simulink model "vidcap_webcam"  (R2018a)
settings: Solver=FixedStepAuto  StartTime=0.0  StopTime=inf  RelTol=1e-3  EnableMultiTasking=on
undefined symbols (not defined in the file): Rec, SDTV, videoinput
libraries: embdlinuxlib x3, simulink x3, visiontextngfix x2, visionstatistics x1, visionconversions x1, imaqlib x1, visionanalysis x1
settings Model: Creator=migue  LastModifiedBy=migue
settings SolverCC: PositivePriorityOrder=on
settings OptimizationCC: EnhancedBackFolding=on  PassReuseOutputArgsAs=Individual arguments  MaxStackSize=64  OptimizeBlockOrder=speed  DifferentSizesBufferReuse=on  OptimizationCustomize=off
settings DebuggingCC: ParameterTunabilityLossMsg=error
settings HardwareCC: ProdBitPerPointer=32  ProdBitPerSizeT=32  ProdBitPerPtrDiffT=32  ProdLargestAtomicInteger=Long  ProdLargestAtomicFloat=Double  ProdWordSize=32  ProdHWDeviceType=ARM Compatible->ARM Cortex
settings SFSimCC: MATLABDynamicMemAlloc=off
settings RTWCC: SystemTargetFile=ert.tlc  HardwareBoard=Raspberry Pi  TLCOptions="-aInlineSetEventsForThisBaseRateFcn=TLC_FALSE -aSuppressMultiTaskScheduler=TLC_FALSE  -aRateBasedStepFcn=0"  TemplateMakefile=ert_default_tmf  GenerateReport=on  Toolchain=GNU GCC Raspberry Pi  BuildConfiguration=Faster Runs  IncludeHyperlinkInReport=on  LaunchReport=on  GenerateTraceInfo=on  GenerateTraceReport=on  GenerateTraceReportSl=on  GenerateTraceReportSf=on  GenerateTraceReportEml=on
settings CodeAppCC: ForceParamTrailComments=on  IgnoreCustomStorageClasses=off  OperatorAnnotations=on  SimulinkDataObjDesc=on  SFDataObjDesc=on  InsertBlockDesc=on
settings ERTTargetCC: SupportVariableSizeSignals=on

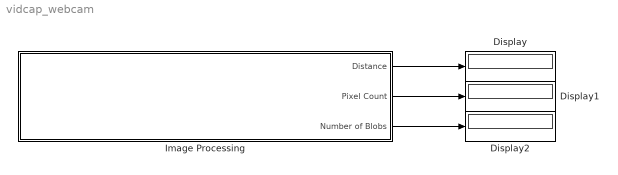
== system vidcap_webcam ==
  Display : Display
  Display1 : Display
  Display2 : Display
  "Image Processing " : Subsystem
  wires:
  "Image Processing "/1(Distance) -> Display/1
  "Image Processing "/2(Pixel Count) -> Display1/1
  "Image Processing "/3(Number of Blobs) -> Display2/1

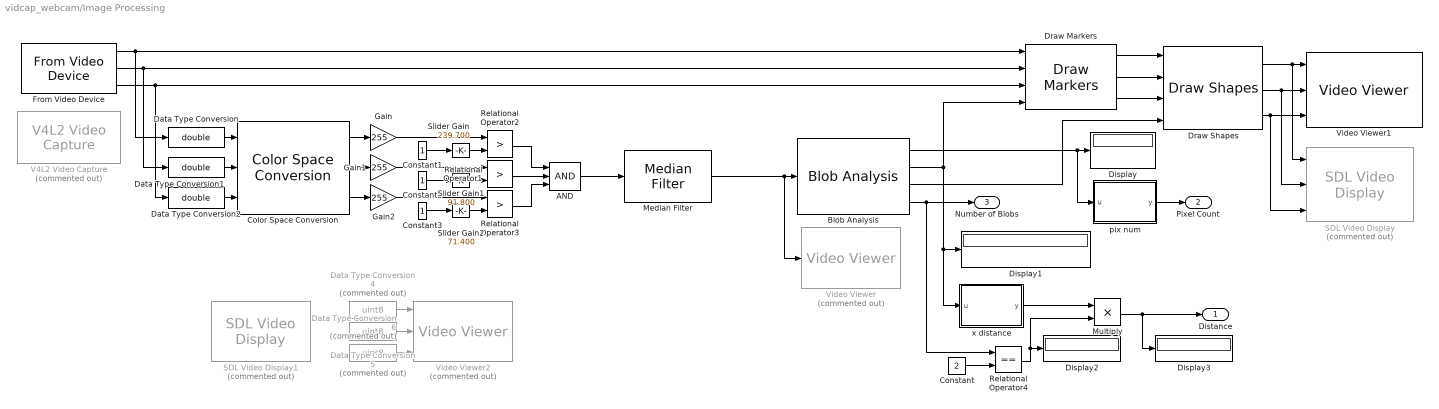
== system vidcap_webcam/Image Processing  ==
  AND : Logic  Inputs=3  IconShape=distinctive  AllPortsSameDT=off  OutDataTypeStr=boolean
  Blob Analysis : visionstatistics/Blob Analysis  Tag=vipblks_row_conv  area=on  centroid=on  bBox=on  majorAxis=off  minorAxis=off  angle=off  eccentricity=off  equivDiameterSq=off  extent=off  perimeter=off  maxBlobs=2  warnIfNumBlobsExceeded=on  isCount=on  useMinArea=on  minArea=2500  useMaxArea=off  maxArea=intmax('uint32')  excludeBorderBlob=off  outDT=double  isOutVarDim=off  isFill=on  fillValues=-1  conn=8  isLabel=off  outputMode=Binary point scaling  outputWordLength=32  outputFracLength=16  firstCoeffMode=Binary point scaling  firstCoeffWordLength=16  firstCoeffFracLength=14  secondCoeffMode=Binary point scaling  secondCoeffWordLength=32  secondCoeffFracLength=16  accumMode=Binary point scaling  accumWordLength=32  accumFracLength=0  prodOutputMode=Binary point scaling  prodOutputWordLength=32  prodOutputFracLength=16  roundingMode=Floor  overflowMode=off
      settings: SourceProductName=Computer Vision System Toolbox
  Color Space Conversion : visionconversions/Color Space  Conversion  conversion=Obsolete  conversionActive=R'G'B' to HSV  wp_str=D65  rec=Rec. 601 (SDTV)  sys=1125/60/2:1  imagePorts=Separate color signals
      settings: SourceProductName=Computer Vision System Toolbox
  Constant : Constant  Value=2
  Constant1 : Constant  OutDataTypeStr=uint8
  Constant2 : Constant  OutDataTypeStr=uint8
  Constant3 : Constant  OutDataTypeStr=uint8
  Data Type Conversion : DataTypeConversion  OutDataTypeStr=double  RndMeth=Simplest  LockScale=on
  Data Type Conversion1 : DataTypeConversion  OutDataTypeStr=double  RndMeth=Simplest  LockScale=on
  Data Type Conversion2 : DataTypeConversion  OutDataTypeStr=double  RndMeth=Simplest  LockScale=on
  Data Type Conversion4 : DataTypeConversion  Commented=on  OutDataTypeStr=uint8
  Data Type Conversion5 : DataTypeConversion  Commented=on  OutDataTypeStr=uint8
  Data Type Conversion6 : DataTypeConversion  Commented=on  OutDataTypeStr=uint8
  Display{,1..3} (4 alike) : Display
  Draw Markers : visiontextngfix/Draw Markers  shape=X-mark  size=5  fill=off  fillClrSource=Specify via dialog  display=White  intensity=200  color=[200 255 100]  opacity=0.6  viewport=Entire image  antialiasing=off  inType=Obsolete  imagePorts=Separate color signals  prodOutputMode=Binary point scaling  prodOutputWordLength=32  prodOutputFracLength=14  memoryMode=Specify word length  memoryWordLength=16  memoryFracLength=15  roundingMode=Floor  overflowMode=off
      settings: SourceProductName=Computer Vision System Toolbox  SourceProductBaseCode=VP
  Draw Shapes : visiontextngfix/Draw Shapes  shape=Rectangles  fill=off  lineWidth=3  fillClrSource=Specify via dialog  display=White  intensity=200  color=[200 255 100]  opacity=0.6  viewport=Entire image  antialiasing=off  inType=Obsolete  imagePorts=Separate color signals  prodOutputMode=Binary point scaling  prodOutputWordLength=32  prodOutputFracLength=14  memoryMode=Specify word length  memoryWordLength=16  memoryFracLength=15  roundingMode=Floor  overflowMode=off
      settings: SourceProductName=Computer Vision System Toolbox
  From Video Device : imaqlib/From Video Device  DeviceMenu=winvideo 1 (HD WebCam)  Device=winvideo 1 (HD WebCam)  ObjConstructor=videoinput('winvideo', 1)  VideoFormatMenu=MJPG_1280x720  VideoFormat=MJPG_1280x720  VideoSource=input1  ROIPosition=[0 0 480 640]  EnableHWTrigger=off  TriggerConfiguration=winvideo 1 (HD WebCam)  SampleTime=1/30  OutputPortsMode=Separate color signals  DataType=single  CanDoHWTrigger=no  ReturnedColorSpace=rgb  BlockHandle=250.0001  ROIWidth=640  ROIHeight=480  ROIColumn=0  ROIRow=0  EngXMLPath=C:\Program Files\MATLAB\R2018a\toolbox\imaq\imaq\private  DevXMLPath=C:\ProgramData\MATLAB\SupportPackages\R2018a\toolbox\imaq\supportpackages\genericvideo\adaptor\win64  EngLibPath=C:\Program Files\MATLAB\R2018a\toolbox\imaq\imaqblks\imaqmex\win64  ColorSpace=rgb  BayerSensorAlignment=grbg
      settings: SourceProductName=Image Acquisition Toolbox
  Gain : Gain  Gain=255
  Gain1 : Gain  Gain=255
  Gain2 : Gain  Gain=255
  Median Filter : visionanalysis/Median Filter  nghbood=[5 5]  outSize=Same as input port I  padType=Constant  padSrc=Specify via dialog  padVal=0  roundingMode=Floor  overflowMode=off
      settings: SourceProductName=Computer Vision System Toolbox  SourceProductBaseCode=VP
  Multiply : Product  OutDataTypeStr=double  LockScale=on
  Relational Operator1 : RelationalOperator  Operator=>  OutDataTypeStr=boolean  RndMeth=Simplest
  Relational Operator2 : RelationalOperator  Operator=>  OutDataTypeStr=boolean  RndMeth=Simplest
  Relational Operator3 : RelationalOperator  Operator=>  OutDataTypeStr=boolean  RndMeth=Simplest
  Relational Operator4 : RelationalOperator  Operator===  OutDataTypeStr=boolean  RndMeth=Simplest
  SDL Video Display : embdlinuxlib/SDL Video Display  Commented=on  pixelFormat=RGB  pixelOrder=Planar  rowMajor=on  blockPlatform=Raspberry Pi
      settings: SourceProductName=Simulink Support Package for Raspberry Pi Hardware  SourceProductBaseCode=RASPPI
  SDL Video Display1 : embdlinuxlib/SDL Video Display  Commented=on  pixelFormat=RGB  pixelOrder=Planar  rowMajor=on  blockPlatform=Raspberry Pi
      settings: SourceProductName=Simulink Support Package for Raspberry Pi Hardware  SourceProductBaseCode=RASPPI
  Slider Gain : simulink/Math Operations/Slider Gain  gain=239.700  low=0  high=255
  Slider Gain1 : simulink/Math Operations/Slider Gain  gain=91.800  low=0  high=255
  Slider Gain2 : simulink/Math Operations/Slider Gain  gain=71.400  low=0  high=255
  V4L2 Video Capture : embdlinuxlib/V4L2 Video Capture  Commented=on  m_devName='/dev/video0'  roi=[0, 0, 640, 480]  imSizeSelection=640x480  imSize=[1280, 720]  pixelFormat=RGB  pixelOrder=Planar  sampleTime=1/10  simOutput=Colorbars  blockPlatform=Raspberry Pi
      settings: SourceProductName=Simulink Support Package for Raspberry Pi Hardware  SourceProductBaseCode=RASPPI
  Video Viewer : VideoViewer  Commented=on  FigPos=[561 735 732 627]
  Video Viewer1 : VideoViewer  imagePorts=separate color signals  FigPos=[3 755 732 627]
  Video Viewer2 : VideoViewer  Commented=on  imagePorts=separate color signals  FigPos=[271 744 732 627]
  pix num : MATLAB Function  TreatAsAtomicUnit=on
  x distance : MATLAB Function  TreatAsAtomicUnit=on
  Distance : Outport
  Pixel Count : Outport  Port=2
  Number of Blobs : Outport  Port=3
  wires:
  Constant1/1 -> Slider Gain/1
  Draw Markers/2 -> Draw Shapes/2
  Draw Shapes/3 -> Video Viewer1/3, SDL Video Display/3
  From Video Device/3 -> Data Type Conversion2/1, Draw Markers/3
  Blob Analysis/3 -> Draw Shapes/4
  Draw Shapes/1 -> SDL Video Display/1, Video Viewer1/1
  Data Type Conversion/1 -> Color Space Conversion/1
  Draw Shapes/2 -> Video Viewer1/2, SDL Video Display/2
  From Video Device/1 -> Draw Markers/1, Data Type Conversion/1
  From Video Device/2 -> Draw Markers/2, Data Type Conversion1/1
  Blob Analysis/1 -> pix num/1(u), Display/1
  Median Filter/1 -> Video Viewer/1, Blob Analysis/1
  Data Type Conversion1/1 -> Color Space Conversion/2
  Blob Analysis/2 -> x distance/1(u), Display1/1, Draw Markers/4
  Draw Markers/1 -> Draw Shapes/1
  Data Type Conversion2/1 -> Color Space Conversion/3
  Draw Markers/3 -> Draw Shapes/3
  Data Type Conversion4/1 -> Video Viewer2/1
  Data Type Conversion5/1 -> Video Viewer2/2
  Data Type Conversion6/1 -> Video Viewer2/3
  Slider Gain/1 -> Relational Operator2/2
  Color Space Conversion/1 -> Gain/1
  Gain/1 -> Relational Operator2/1
  Color Space Conversion/2 -> Gain1/1
  Color Space Conversion/3 -> Gain2/1
  Gain1/1 -> Relational Operator1/1
  Slider Gain1/1 -> Relational Operator1/2
  Constant2/1 -> Slider Gain1/1
  Gain2/1 -> Relational Operator3/1
  Slider Gain2/1 -> Relational Operator3/2
  Constant3/1 -> Slider Gain2/1
  Relational Operator2/1 -> AND/1
  Relational Operator1/1 -> AND/2
  Relational Operator3/1 -> AND/3
  AND/1 -> Median Filter/1
  pix num/1(y) -> Pixel Count/1
  Multiply/1 -> Display3/1, Distance/1
  x distance/1(y) -> Multiply/1
  Blob Analysis/4 -> Number of Blobs/1, Relational Operator4/1
  Constant/1 -> Relational Operator4/2
  Relational Operator4/1 -> Display2/1, Multiply/2

== matlab function vidcap_webcam/Image Processing /pix num ==
  data: u input; y output
function y = area(u)

y = u(1) + u(2);

== matlab function vidcap_webcam/Image Processing /x distance ==
  data: u input; y output
function y = dist(u)

y = abs(u(2,1) - u(1,1));
